simulink model "math_operators_simulink"  (R2022a)
settings: Solver=VariableStepAuto  StartTime=0.0  StopTime=10.0  RelTol=1e-3
libraries: simulink x1
settings Model: Creator=Home computer  LastModifiedBy=Home computer

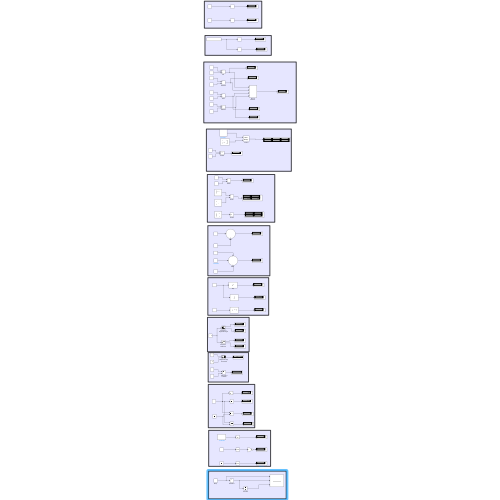
[thumbnail: Simulink's stored preview of the top-level diagram]
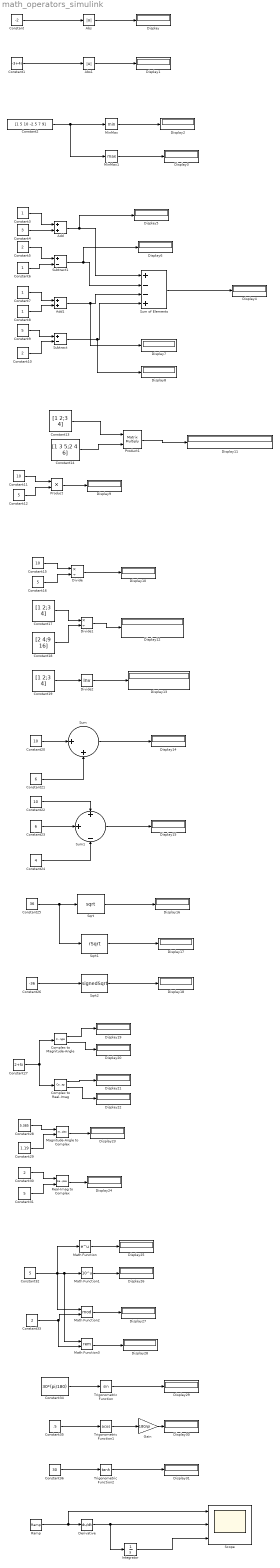
== system math_operators_simulink ==
  Abs : Abs  SaturateOnIntegerOverflow=off
  Abs1 : Abs  SaturateOnIntegerOverflow=off
  Add : Sum
  Add1 : Sum
  Complex to Magnitude-Angle : ComplexToMagnitudeAngle
  Complex to Real-Imag : ComplexToRealImag
  Constant : Constant  Value=-2
  Constant1 : Constant  Value=-3+4i
  Constant{5,10,30,33} (4 alike) : Constant  Value=2
  Constant{11,15,20,22} (4 alike) : Constant  Value=10
  Constant{9,12,16,31..32} (5 alike) : Constant  Value=5
  Constant13 : Constant  Value=[1 2;3 4]
  Constant14 : Constant  Value=[1 3 5;2 4 6]
  Constant17 : Constant  Value=[1 2;3 4]
  Constant18 : Constant  Value=[2 4;9 16]
  Constant19 : Constant  Value=[1 2;3 4]
  Constant2 : Constant  Value=[1 5 10 -2.5 7 9]
  Constant21 : Constant  Value=6
  Constant23 : Constant  Value=6
  Constant24 : Constant  Value=4
  Constant25 : Constant  Value=36
  Constant26 : Constant  Value=-36
  Constant27 : Constant  Value=2+5i
  Constant28 : Constant  Value=5.385
  Constant29 : Constant  Value=1.19
  Constant{3,6..8} (4 alike) : Constant
  Constant34 : Constant  Value=30*(pi/180)
  Constant35 : Constant  Value=.5
  Constant36 : Constant  Value=30
  Constant4 : Constant  Value=3
  Derivative : Derivative
  Display{,1..31} (32 alike) : Display
  Divide : Product  Inputs=*/
  Divide1 : Product  Inputs=*/
  Divide2 : Product  Inputs=/  Multiplication=Matrix(*)
  Gain : Gain  Gain=180/pi
  Integrator : Integrator
  Magnitude-Angle to Complex : MagnitudeAngleToComplex
  Math Function : Math
  Math Function1 : Math  Operator=10^u
  Math Function2 : Math  Operator=mod
  Math Function3 : Math  Operator=rem
  MinMax : MinMax
  MinMax1 : MinMax  Function=max
  Product : Product
  Product1 : Product  Multiplication=Matrix(*)
  Ramp : simulink/Sources/Ramp  slope=1  start=0  InitialOutput=0
  Real-Imag to Complex : RealImagToComplex
  Scope : Scope  NumInputPorts=3
  Sqrt : Sqrt
  Sqrt1 : Sqrt  Operator=rSqrt
  Sqrt2 : Sqrt  Operator=signedSqrt
  Subtract : Sum  Inputs=+-
  Subtract1 : Sum  Inputs=+-
  Sum : Sum  Inputs=|++
  Sum of Elements : Sum  Inputs=+--+
  Sum1 : Sum  Inputs=+|+|-
  Trigonometric Function : Trigonometry
  Trigonometric Function1 : Trigonometry  Operator=acos
  Trigonometric Function2 : Trigonometry  Operator=tanh
  wires:
  Constant/1 -> Abs/1
  Abs/1 -> Display/1
  Constant1/1 -> Abs1/1
  Abs1/1 -> Display1/1
  Constant2/1 -> MinMax1/1, MinMax/1
  MinMax/1 -> Display2/1
  MinMax1/1 -> Display3/1
  Add/1 -> Display5/1, Sum of Elements/1
  Subtract1/1 -> Display6/1, Sum of Elements/2
  Add1/1 -> Display7/1, Sum of Elements/3
  Subtract/1 -> Display8/1, Sum of Elements/4
  Constant3/1 -> Add/1
  Constant4/1 -> Add/2
  Constant5/1 -> Subtract1/1
  Constant6/1 -> Subtract1/2
  Constant7/1 -> Add1/1
  Constant8/1 -> Add1/2
  Constant9/1 -> Subtract/1
  Constant10/1 -> Subtract/2
  Sum of Elements/1 -> Display4/1
  Constant11/1 -> Product/1
  Constant12/1 -> Product/2
  Product/1 -> Display9/1
  Divide/1 -> Display10/1
  Constant13/1 -> Product1/1
  Constant14/1 -> Product1/2
  Product1/1 -> Display11/1
  Constant16/1 -> Divide/2
  Constant15/1 -> Divide/1
  Constant17/1 -> Divide1/1
  Constant18/1 -> Divide1/2
  Divide1/1 -> Display12/1
  Constant19/1 -> Divide2/1
  Divide2/1 -> Display13/1
  Constant20/1 -> Sum/1
  Constant21/1 -> Sum/2
  Constant22/1 -> Sum1/1
  Constant23/1 -> Sum1/2
  Constant24/1 -> Sum1/3
  Sum/1 -> Display14/1
  Sum1/1 -> Display15/1
  Constant25/1 -> Sqrt1/1, Sqrt/1
  Sqrt/1 -> Display16/1
  Sqrt1/1 -> Display17/1
  Sqrt2/1 -> Display18/1
  Constant26/1 -> Sqrt2/1
  Constant27/1 -> Complex to Real-Imag/1, Complex to Magnitude-Angle/1
  Complex to Magnitude-Angle/1 -> Display19/1
  Complex to Magnitude-Angle/2 -> Display20/1
  Complex to Real-Imag/1 -> Display21/1
  Complex to Real-Imag/2 -> Display22/1
  Constant30/1 -> Real-Imag to Complex/1
  Constant31/1 -> Real-Imag to Complex/2
  Constant29/1 -> Magnitude-Angle to Complex/2
  Constant28/1 -> Magnitude-Angle to Complex/1
  Magnitude-Angle to Complex/1 -> Display23/1
  Real-Imag to Complex/1 -> Display24/1
  Constant32/1 -> Math Function2/1, Math Function3/1, Math Function1/1, Math Function/1
  Constant33/1 -> Math Function3/2, Math Function2/2
  Math Function/1 -> Display25/1
  Math Function1/1 -> Display26/1
  Math Function2/1 -> Display27/1
  Math Function3/1 -> Display28/1
  Constant34/1 -> Trigonometric Function/1
  Constant35/1 -> Trigonometric Function1/1
  Constant36/1 -> Trigonometric Function2/1
  Trigonometric Function1/1 -> Gain/1
  Trigonometric Function/1 -> Display29/1
  Gain/1 -> Display30/1
  Trigonometric Function2/1 -> Display31/1
  Ramp/1 -> Scope/1, Derivative/1
  Derivative/1 -> Integrator/1, Scope/2
  Integrator/1 -> Scope/3
